simulink model "simulation_model"  (R2024b)
settings: Solver=VariableStepAuto  StartTime=0.0  StopTime=100  MaxStep=1/60  RelTol=1e-3  EnableMultiTasking=on
values from neighbouring files (symbols this model uses):
  c_f = c_f*Cb    [fun00_GFL_pu_2_normial.m]    (also in fun00_GFM_pu_2_normial.m)
  fb = 60    [case_data.m]    (also in sim_m_case1.m; sim_m_case1_bench.m; sim_m_case2.m; sim_m_case2_bench.m)
  ki_i = ki_i_pu*Vb_p_ph/Ib_p_ph    [fun00_GFL_pu_2_normial.m]    (also in fun00_GFM_pu_2_normial.m)
  ki_p = ki_p_pu/Sb*Ib_p_ph    [fun00_GFL_pu_2_normial.m]
  ki_pll = ki_pll/Vb_p_ph    [fun00_GFL_pu_2_normial.m]
  ki_q = ki_q_pu/Sb*Ib_p_ph    [fun00_GFL_pu_2_normial.m]
  kp_i = kp_i_pu*Vb_p_ph/Ib_p_ph    [fun00_GFL_pu_2_normial.m]    (also in fun00_GFM_pu_2_normial.m)
  kp_p = kp_p_pu/Sb*Ib_p_ph    [fun00_GFL_pu_2_normial.m]
  kp_pll = kp_pll/Vb_p_ph    [fun00_GFL_pu_2_normial.m]
  kp_q = kp_q_pu/Sb*Ib_p_ph    [fun00_GFL_pu_2_normial.m]
  l_f = l_f*Lb    [fun00_GFL_pu_2_normial.m]    (also in fun00_GFM_pu_2_normial.m)
  line = mpc.line    [sim_m_case1.m]    (also in sim_m_case1_bench.m; sim_m_case2.m = mpc.line*1.1; sim_m_case2_bench.m = mpc.line*1.1; sim_m_case2_sparse.m = mpc.line*1.1)
  pset = p_set_pu*Sb    [fun00_GFL_pu_2_normial.m]
  qset = q_set_pu*Sb    [fun00_GFL_pu_2_normial.m]
  r_f = r_f*Zb    [fun00_GFL_pu_2_normial.m]    (also in fun00_GFM_pu_2_normial.m)
  Sb = 100*10^6    (= 100000000)    [sim_m_case1.m]    (also in sim_m_case1_bench.m; sim_m_case2.m; sim_m_case2_bench.m; sim_m_case2_sparse.m)
  t_gfl = 35    [sim_m_case1.m]    (also in sim_m_case1_bench.m = 30; sim_m_case2.m; sim_m_case2_bench.m = 30; sim_m_case2_sparse.m)
  t_gfm = 30    [sim_m_case1.m]    (also in sim_m_case1_bench.m; sim_m_case2.m; sim_m_case2_bench.m; sim_m_case2_sparse.m)
  trans_l = mpc.trans_l    [sim_m_case1.m]    (also in sim_m_case1_bench.m; sim_m_case2.m; sim_m_case2_bench.m; sim_m_case2_sparse.m)
  Vb_gfm = 20*10^3    (= 20000)    [sim_m_case1.m]    (also in sim_m_case1_bench.m; sim_m_case2.m; sim_m_case2_bench.m; sim_m_case2_sparse.m)
  Vdc = 3*Vb_p_ph    [fun00_GFL_pu_2_normial.m]    (also in fun00_GFM_pu_2_normial.m)
  wb = 2*pi*fb    (= 376.991118431)    [case_data.m]    (also in sim_m_case1.m; sim_m_case1_bench.m; sim_m_case2.m; sim_m_case2_bench.m)
undefined symbols (not defined in the file or in its folder): c_f_gfm, d_gfl, D_p_gfm, D_p_gfm_s, D_q_gfm, DiscIntNeverNeededParam, Init, Init_GFL, J_gfm, ki_i_gfm, ki_pll_s, ki_vc_gfm, kp_i_gfm, kp_pll_s, kp_vc_gfm, l_f_gfm, P_set_gfm, Q_set_gfm, r_f_gfm, Vb, Vdc_gfm, VSM
libraries: spsThreePhaseVIMeasurementLib x52, spsabctodq0Lib x48, slpidlib x42, spsThreePhaseSeriesRLCBranchLib x27, spsFirstOrderFilterLib x16, spsThreePhaseTransformerTwoWindingsLib x9, spsGroundLib x9, spsPowerPositiveSequenceLib x9, spsdq0toabcLib x9, spsUniversalBridgeLib x9, spsDCVoltageSourceLib x9, spsThreePhaseParallelRLCLoadLib x6
(part 3 of 8)

== system simulation_model/Area 2/INVERTER 6/GFL6 ==
  Cf : spsThreePhaseSeriesRLCBranchLib/Three-Phase Series RLC Branch  Commented=on  LConnTagsString=A|B|C  RConnTagsString=A|B|C  BranchType=C  Resistance=0.1  Inductance=1e-3  Capacitance=RLC_Filter(3)  Measurements=None
  Constant : Constant  Value=Pref
  Constant1 : Constant  Value=Qref
  Display : Display
  Display1 : Display
  Gain : Gain  Gain=1/(Vnom*sqrt(2/3))
  Gain1 : Gain  Gain=1/Sb
  Gain2 : Gain  Gain=1/2/pi/fb
  Gain3 : Gain  Gain=1/Sb
  Ground : spsGroundLib/Ground  Commented=on  LConnTagsString=a
  Measurement : Subsystem
      mask DialogControl ParameterGroupVar Prompt: 参数
  PLL : Subsystem
      mask DialogControl ParameterGroupVar Prompt: 参数
  Subsystem3 : Subsystem
      mask DialogControl ParameterGroupVar Prompt: 参数
  Subsystem4 : Subsystem  mask{Voltage_P=Voltage_P, Voltage_I=Voltage_I, Current_P=Current_P, Current_I=Current_I, Power_P=Power_P, Power_I=Power_I, kf=kf, Dgfl=D_gfl}
      mask prompts: Voltage_P "Voltage Proportional Coefficient"; Voltage_I "Voltage Integral Coefficient"; Current_P "Current Proportional Coefficient"; Current_I "Current Integral Coefficient"; Power_P "Power Proportional Coefficient"; Power_I "Power Integral Coefficient"; kf "Feedforward Coeffcient"; Dgfl "Damping"
      mask DialogControl ParameterGroupVar Prompt: Controller Parameter
  Three-Phase Series RLC Branch : spsThreePhaseSeriesRLCBranchLib/Three-Phase Series RLC Branch  LConnTagsString=A|B|C  RConnTagsString=A|B|C  BranchType=RL  Resistance=RLC_Filter(1)  Inductance=RLC_Filter(2)  Capacitance=1e-6  Measurements=None
  Three-Phase V-I Measurement : spsThreePhaseVIMeasurementLib/Three-Phase V-I Measurement  VoltageMeasurement=phase-to-ground  SetLabelV=off  LabelV=Vabc_s2  Vpu=off  VpuLL=off  CurrentMeasurement=yes  SetLabelI=off  LabelI=Iabc_s2  Ipu=off  Pbase=Pnom  Vbase=Vnom  OutputType=Complex  PhasorSimulation=off  PSBequivalent=0
  Three-Phase V-I Measurement1 : spsThreePhaseVIMeasurementLib/Three-Phase V-I Measurement  VoltageMeasurement=phase-to-ground  SetLabelV=off  LabelV=Vabc_s1  Vpu=off  VpuLL=off  CurrentMeasurement=yes  SetLabelI=off  LabelI=Iabc_s1  Ipu=off  Pbase=Pnom  Vbase=Vnom  OutputType=Complex  PhasorSimulation=off  PSBequivalent=0
  Three-Phase V-I Measurement2 : spsThreePhaseVIMeasurementLib/Three-Phase V-I Measurement  VoltageMeasurement=phase-to-ground  SetLabelV=off  LabelV=Vabc_s0  Vpu=off  VpuLL=off  CurrentMeasurement=yes  SetLabelI=off  LabelI=Iabc_s0  Ipu=off  Pbase=Pnom  Vbase=Vnom  OutputType=Complex  PhasorSimulation=off  PSBequivalent=0
  Three-Phase V-I Measurement3 : spsThreePhaseVIMeasurementLib/Three-Phase V-I Measurement  VoltageMeasurement=phase-to-ground  SetLabelV=off  LabelV=Vabc_s2  Vpu=off  VpuLL=off  CurrentMeasurement=yes  SetLabelI=off  LabelI=Iabc_s2  Ipu=off  Pbase=Pnom  Vbase=Vnom  OutputType=Complex  PhasorSimulation=off  PSBequivalent=0
  Universal Bridge : spsUniversalBridgeLib/Universal Bridge  Arms=3  SnubberResistance=1e5  SnubberCapacitance=inf  Device=Average-model based VSC  Ron=1e-3  Lon=0  ForwardVoltages="[  0  0  ]"  ForwardVoltage=0  GTOparameters=[ 10e-6 , 20e-6 ]  IGBTparameters=[ 1e-6 , 2e-6 ]  Measurements=None  Measurements_2=None  converterType=Rectifier
  Vdc : spsDCVoltageSourceLib/DC Voltage Source  Amplitude=Vdc_nom  Measurements=None
  Vrms : Scope
  a : PMIOPort  Side=Right
  b : PMIOPort  Port=2  Side=Right
  c : PMIOPort  Port=3  Side=Right
  P : Outport
  Omega : Outport  Port=2
  Vabs : Outport  Port=3
  theta_t : Outport  Port=4
  Q : Outport  Port=5
  theta_0 : Outport  Port=6
  wires:
  Measurement/5(Vrms) -> Gain/1, Vrms/1
  Measurement/2(Q) -> Gain1/1, [Q]
  Measurement/3(Vodq) -> [Vodq]
  Measurement/4(Icdq) -> [Icdq]
  [Vabc_s0] -> Measurement/1(Vabc_s0)
  [theta] -> Measurement/4(theta)
  [Iabc_s2] -> Measurement/3(Iabc_s2)
  [Iabc_s0] -> Measurement/2(Iabc_s0)
  [VSG_Uref] -> Universal Bridge/1
  [Vabc_s0] -> PLL/1(Vodq)
  Three-Phase V-I Measurement3/1 -> Subsystem3/1(Vabc)
  Three-Phase V-I Measurement3/2 -> Subsystem3/2(Iabc)
  Subsystem3/1(Vdq0) -> Display/1
  Subsystem3/2(Idq0) -> Display1/1
  PLL/2(theta) -> [theta]
  [Icdq] -> Subsystem4/2(Icdq)
  [Vodq] -> Subsystem4/1(Vodq)
  [theta] -> Subsystem4/3(theta)
  Subsystem4/1(VSG_Uref) -> [VSG_Uref]
  Three-Phase V-I Measurement/1 -> [Vabc_s2]
  Three-Phase V-I Measurement/2 -> [Iabc_s2]
  Three-Phase V-I Measurement2/1 -> [Vabc_s0]
  Three-Phase V-I Measurement2/2 -> [Iabc_s0]
  Three-Phase V-I Measurement1/2 -> [Iabc_s1]
  Three-Phase V-I Measurement1/1 -> [Vabc_s1]
  [P] -> Subsystem4/5(P)
  Constant/1 -> Subsystem4/4(pset)
  Constant1/1 -> Subsystem4/6(qset)
  [theta] -> Subsystem3/3(theta)
  Measurement/1(P) -> Gain3/1, [P]
  PLL/3(Omega) -> [omega], Gain2/1
  Gain/1 -> Vabs/1
  Gain2/1 -> Omega/1
  Gain3/1 -> P/1
  PLL/1(theta_GFL) -> theta_t/1
  Gain1/1 -> Q/1
  PLL/4(theta_0) -> theta_0/1
  [Q] -> Subsystem4/7(Q)
  [omega] -> Subsystem4/8(Omega)
  connections:
  Three-Phase V-I Measurement2/LConn2 -- Cf/LConn2 -- Three-Phase V-I Measurement1/RConn2
  Three-Phase V-I Measurement2/LConn1 -- Cf/LConn1 -- Three-Phase V-I Measurement1/RConn1
  Three-Phase V-I Measurement2/LConn3 -- Cf/LConn3 -- Three-Phase V-I Measurement1/RConn3
  Three-Phase V-I Measurement1/LConn2 -- Three-Phase Series RLC Branch/RConn2
  Three-Phase V-I Measurement1/LConn1 -- Three-Phase Series RLC Branch/RConn1
  Universal Bridge/RConn2 -- Vdc/LConn1
  Vdc/RConn1 -- Universal Bridge/RConn1
  Three-Phase V-I Measurement/LConn3 -- Universal Bridge/LConn3
  Three-Phase V-I Measurement/LConn2 -- Universal Bridge/LConn2
  Three-Phase V-I Measurement/LConn1 -- Universal Bridge/LConn1
  Three-Phase V-I Measurement1/LConn3 -- Three-Phase Series RLC Branch/RConn3
  Three-Phase V-I Measurement2/RConn1 -- a/RConn1
  Three-Phase V-I Measurement2/RConn2 -- b/RConn1
  Three-Phase V-I Measurement2/RConn3 -- c/RConn1
  Three-Phase V-I Measurement3/RConn1 -- Three-Phase Series RLC Branch/LConn1
  Three-Phase Series RLC Branch/LConn2 -- Three-Phase V-I Measurement3/RConn2
  Three-Phase Series RLC Branch/LConn3 -- Three-Phase V-I Measurement3/RConn3
  Three-Phase V-I Measurement3/LConn1 -- Three-Phase V-I Measurement/RConn1
  Three-Phase V-I Measurement3/LConn2 -- Three-Phase V-I Measurement/RConn2
  Three-Phase V-I Measurement3/LConn3 -- Three-Phase V-I Measurement/RConn3
  Ground/LConn1 -- Cf/RConn2 -- Cf/RConn1 -- Cf/RConn3

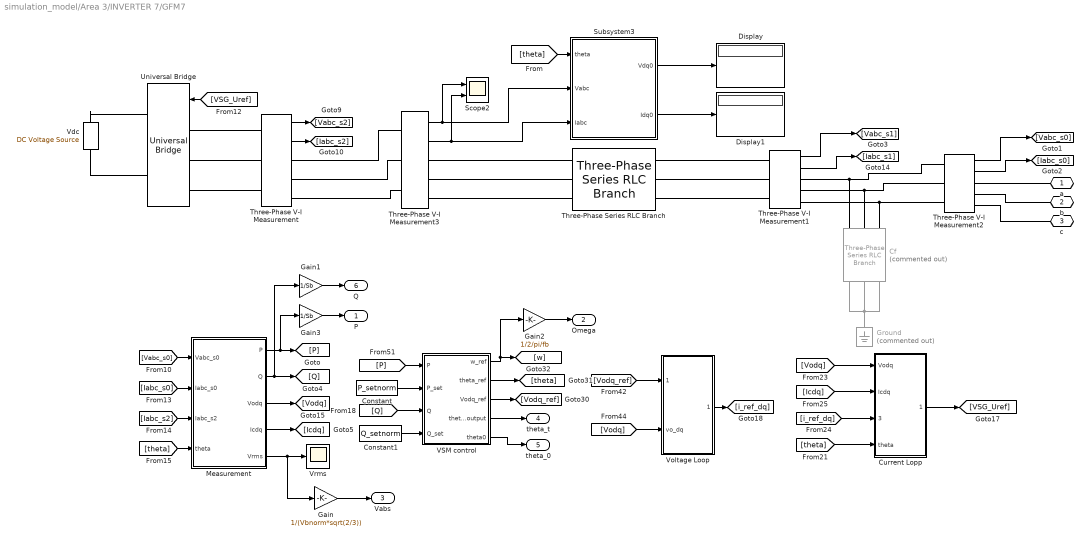
== system simulation_model/Area 3/INVERTER 7/GFM7 ==
  Cf : spsThreePhaseSeriesRLCBranchLib/Three-Phase Series RLC Branch  Commented=on  LConnTagsString=A|B|C  RConnTagsString=A|B|C  BranchType=C  Resistance=0.1  Inductance=1e-3  Capacitance=RLCnorm(3)  Measurements=None
  Constant : Constant  Value=P_setnorm
  Constant1 : Constant  Value=Q_setnorm
  Current Lopp : Subsystem  mask{Current_P=Current_P, Current_I=Current_I}
      mask prompts: Current_P "Current Proportional Coefficient"; Current_I "Current Integral Coefficient"
  Display : Display
  Display1 : Display
  Gain : Gain  Gain=1/(Vbnorm*sqrt(2/3))
  Gain1 : Gain  Gain=1/Sb
  Gain2 : Gain  Gain=1/2/pi/fb
  Gain3 : Gain  Gain=1/Sb
  Ground : spsGroundLib/Ground  Commented=on  LConnTagsString=a
  Measurement : Subsystem
      mask DialogControl ParameterGroupVar Prompt: 参数
  Scope2 : Scope  NumInputPorts=2
  Subsystem3 : Subsystem
      mask DialogControl ParameterGroupVar Prompt: 参数
  Three-Phase Series RLC Branch : spsThreePhaseSeriesRLCBranchLib/Three-Phase Series RLC Branch  LConnTagsString=A|B|C  RConnTagsString=A|B|C  BranchType=RL  Resistance=RLCnorm(1)  Inductance=RLCnorm(2)  Capacitance=1e-6  Measurements=None
  Three-Phase V-I Measurement : spsThreePhaseVIMeasurementLib/Three-Phase V-I Measurement  VoltageMeasurement=phase-to-ground  SetLabelV=off  LabelV=Vabc_s2  Vpu=off  VpuLL=off  CurrentMeasurement=yes  SetLabelI=off  LabelI=Iabc_s2  Ipu=off  Pbase=Pnom  Vbase=Vnom  OutputType=Complex  PhasorSimulation=off  PSBequivalent=0
  Three-Phase V-I Measurement1 : spsThreePhaseVIMeasurementLib/Three-Phase V-I Measurement  VoltageMeasurement=phase-to-ground  SetLabelV=off  LabelV=Vabc_s1  Vpu=off  VpuLL=off  CurrentMeasurement=yes  SetLabelI=off  LabelI=Iabc_s1  Ipu=off  Pbase=Pnom  Vbase=Vnom  OutputType=Complex  PhasorSimulation=off  PSBequivalent=0
  Three-Phase V-I Measurement2 : spsThreePhaseVIMeasurementLib/Three-Phase V-I Measurement  VoltageMeasurement=phase-to-ground  SetLabelV=off  LabelV=Vabc_s0  Vpu=off  VpuLL=off  CurrentMeasurement=yes  SetLabelI=off  LabelI=Iabc_s0  Ipu=off  Pbase=Pnom  Vbase=Vnom  OutputType=Complex  PhasorSimulation=off  PSBequivalent=0
  Three-Phase V-I Measurement3 : spsThreePhaseVIMeasurementLib/Three-Phase V-I Measurement  VoltageMeasurement=phase-to-ground  SetLabelV=off  LabelV=Vabc_s2  Vpu=off  VpuLL=off  CurrentMeasurement=yes  SetLabelI=off  LabelI=Iabc_s2  Ipu=off  Pbase=Pnom  Vbase=Vnom  OutputType=Complex  PhasorSimulation=off  PSBequivalent=0
  Universal Bridge : spsUniversalBridgeLib/Universal Bridge  Arms=3  SnubberResistance=1e5  SnubberCapacitance=inf  Device=Average-model based VSC  Ron=1e-3  Lon=0  ForwardVoltages="[  0  0  ]"  ForwardVoltage=0  GTOparameters=[ 10e-6 , 20e-6 ]  IGBTparameters=[ 1e-6 , 2e-6 ]  Measurements=None  Measurements_2=None  converterType=Rectifier
  VSM control : Subsystem  mask{J=Jnorm, Dp=Dpnorm, Dq=Dqnorm}
      mask prompts: J "Inertia"; Dp "Damping"; Dq "Reactive Droop"
  Vdc : spsDCVoltageSourceLib/DC Voltage Source  Amplitude=Vdcnorm  Measurements=None
  Voltage Loop : Subsystem  mask{Voltage_P=Voltage_P, Voltage_I=Voltage_I}
      mask prompts: Voltage_P "Voltage Proportional Gain"; Voltage_I "Voltage Integral Gain"
  Vrms : Scope
  a : PMIOPort  Side=Right
  b : PMIOPort  Port=2  Side=Right
  c : PMIOPort  Port=3  Side=Right
  P : Outport
  Omega : Outport  Port=2
  Vabs : Outport  Port=3
  theta_t : Outport  Port=4
  theta_0 : Outport  Port=5
  Q : Outport  Port=6
  wires:
  [Vodq_ref] -> Voltage Loop/1(v_ref_dq)
  [Vodq] -> Voltage Loop/2(vo_dq)
  VSM control/2(theta_ref) -> [theta]
  Constant/1 -> VSM control/2(P_set)
  [P] -> VSM control/1(P)
  [Q] -> VSM control/3(Q)
  Three-Phase V-I Measurement1/2 -> [Iabc_s1]
  [VSG_Uref] -> Universal Bridge/1
  Subsystem3/1(Vdq0) -> Display/1
  Three-Phase V-I Measurement2/1 -> [Vabc_s0]
  Three-Phase V-I Measurement/2 -> [Iabc_s2]
  Three-Phase V-I Measurement3/2 -> Scope2/2, Subsystem3/3(Iabc)
  Subsystem3/2(Idq0) -> Display1/1
  Three-Phase V-I Measurement/1 -> [Vabc_s2]
  [theta] -> Subsystem3/1(theta)
  Three-Phase V-I Measurement2/2 -> [Iabc_s0]
  Three-Phase V-I Measurement3/1 -> Scope2/1, Subsystem3/2(Vabc)
  Three-Phase V-I Measurement1/1 -> [Vabc_s1]
  [Vabc_s0] -> Measurement/1(Vabc_s0)
  Measurement/5(Vrms) -> Gain/1, Vrms/1
  Measurement/2(Q) -> Gain1/1, [Q]
  Measurement/4(Icdq) -> [Icdq]
  Measurement/1(P) -> Gain3/1, [P]
  Measurement/3(Vodq) -> [Vodq]
  [theta] -> Measurement/4(theta)
  [Iabc_s2] -> Measurement/3(Iabc_s2)
  [Iabc_s0] -> Measurement/2(Iabc_s0)
  VSM control/3(Vodq_ref) -> [Vodq_ref]
  [Icdq] -> Current Lopp/2(Icdq)
  Current Lopp/1(VSG_Uref) -> [VSG_Uref]
  [Vodq] -> Current Lopp/1(Vodq)
  [theta] -> Current Lopp/4(theta)
  Voltage Loop/1(i_ref_dq) -> [i_ref_dq]
  [i_ref_dq] -> Current Lopp/3(i_ref_dq)
  Constant1/1 -> VSM control/4(Q_set)
  Gain/1 -> Vabs/1
  Gain3/1 -> P/1
  Gain2/1 -> Omega/1
  VSM control/1(w_ref) -> Gain2/1, [w]
  VSM control/4(theta_output) -> theta_t/1
  VSM control/5(theta0) -> theta_0/1
  Gain1/1 -> Q/1
  connections:
  Three-Phase V-I Measurement2/LConn1 -- Cf/LConn1 -- Three-Phase V-I Measurement1/RConn1
  Three-Phase V-I Measurement2/LConn2 -- Cf/LConn2 -- Three-Phase V-I Measurement1/RConn2
  Three-Phase V-I Measurement2/LConn3 -- Cf/LConn3 -- Three-Phase V-I Measurement1/RConn3
  Three-Phase V-I Measurement3/LConn1 -- Three-Phase V-I Measurement/RConn1
  Three-Phase V-I Measurement1/LConn3 -- Three-Phase Series RLC Branch/RConn3
  Three-Phase V-I Measurement2/RConn2 -- b/RConn1
  Three-Phase V-I Measurement/LConn3 -- Universal Bridge/LConn3
  Three-Phase V-I Measurement/LConn1 -- Universal Bridge/LConn1
  Vdc/RConn1 -- Universal Bridge/RConn1
  Three-Phase V-I Measurement2/RConn1 -- a/RConn1
  Three-Phase Series RLC Branch/LConn3 -- Three-Phase V-I Measurement3/RConn3
  Three-Phase V-I Measurement/LConn2 -- Universal Bridge/LConn2
  Three-Phase Series RLC Branch/LConn2 -- Three-Phase V-I Measurement3/RConn2
  Three-Phase V-I Measurement2/RConn3 -- c/RConn1
  Three-Phase V-I Measurement1/LConn1 -- Three-Phase Series RLC Branch/RConn1
  Three-Phase V-I Measurement3/RConn1 -- Three-Phase Series RLC Branch/LConn1
  Universal Bridge/RConn2 -- Vdc/LConn1
  Three-Phase V-I Measurement3/LConn3 -- Three-Phase V-I Measurement/RConn3
  Three-Phase V-I Measurement3/LConn2 -- Three-Phase V-I Measurement/RConn2
  Three-Phase V-I Measurement1/LConn2 -- Three-Phase Series RLC Branch/RConn2
  Cf/RConn3 -- Ground/LConn1 -- Cf/RConn2 -- Cf/RConn1

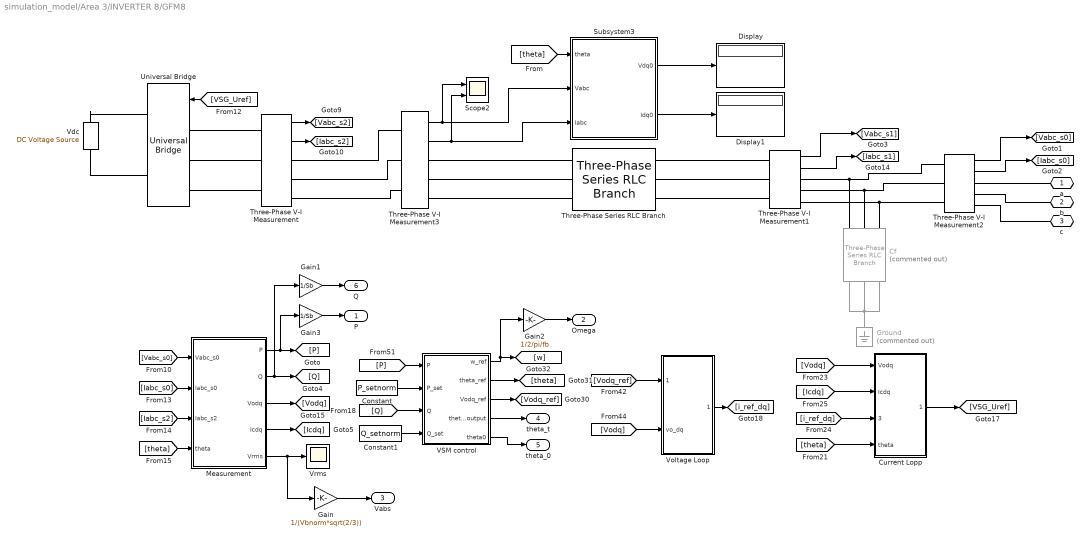
== system simulation_model/Area 3/INVERTER 8/GFM8 ==
  Cf : spsThreePhaseSeriesRLCBranchLib/Three-Phase Series RLC Branch  Commented=on  LConnTagsString=A|B|C  RConnTagsString=A|B|C  BranchType=C  Resistance=0.1  Inductance=1e-3  Capacitance=RLCnorm(3)  Measurements=None
  Constant : Constant  Value=P_setnorm
  Constant1 : Constant  Value=Q_setnorm
  Current Lopp : Subsystem  mask{Current_P=Current_P, Current_I=Current_I}
      mask prompts: Current_P "Current Proportional Coefficient"; Current_I "Current Integral Coefficient"
  Display : Display
  Display1 : Display
  Gain : Gain  Gain=1/(Vbnorm*sqrt(2/3))
  Gain1 : Gain  Gain=1/Sb
  Gain2 : Gain  Gain=1/2/pi/fb
  Gain3 : Gain  Gain=1/Sb
  Ground : spsGroundLib/Ground  Commented=on  LConnTagsString=a
  Measurement : Subsystem
      mask DialogControl ParameterGroupVar Prompt: 参数
  Scope2 : Scope  NumInputPorts=2
  Subsystem3 : Subsystem
      mask DialogControl ParameterGroupVar Prompt: 参数
  Three-Phase Series RLC Branch : spsThreePhaseSeriesRLCBranchLib/Three-Phase Series RLC Branch  LConnTagsString=A|B|C  RConnTagsString=A|B|C  BranchType=RL  Resistance=RLCnorm(1)  Inductance=RLCnorm(2)  Capacitance=1e-6  Measurements=None
  Three-Phase V-I Measurement : spsThreePhaseVIMeasurementLib/Three-Phase V-I Measurement  VoltageMeasurement=phase-to-ground  SetLabelV=off  LabelV=Vabc_s2  Vpu=off  VpuLL=off  CurrentMeasurement=yes  SetLabelI=off  LabelI=Iabc_s2  Ipu=off  Pbase=Pnom  Vbase=Vnom  OutputType=Complex  PhasorSimulation=off  PSBequivalent=0
  Three-Phase V-I Measurement1 : spsThreePhaseVIMeasurementLib/Three-Phase V-I Measurement  VoltageMeasurement=phase-to-ground  SetLabelV=off  LabelV=Vabc_s1  Vpu=off  VpuLL=off  CurrentMeasurement=yes  SetLabelI=off  LabelI=Iabc_s1  Ipu=off  Pbase=Pnom  Vbase=Vnom  OutputType=Complex  PhasorSimulation=off  PSBequivalent=0
  Three-Phase V-I Measurement2 : spsThreePhaseVIMeasurementLib/Three-Phase V-I Measurement  VoltageMeasurement=phase-to-ground  SetLabelV=off  LabelV=Vabc_s0  Vpu=off  VpuLL=off  CurrentMeasurement=yes  SetLabelI=off  LabelI=Iabc_s0  Ipu=off  Pbase=Pnom  Vbase=Vnom  OutputType=Complex  PhasorSimulation=off  PSBequivalent=0
  Three-Phase V-I Measurement3 : spsThreePhaseVIMeasurementLib/Three-Phase V-I Measurement  VoltageMeasurement=phase-to-ground  SetLabelV=off  LabelV=Vabc_s2  Vpu=off  VpuLL=off  CurrentMeasurement=yes  SetLabelI=off  LabelI=Iabc_s2  Ipu=off  Pbase=Pnom  Vbase=Vnom  OutputType=Complex  PhasorSimulation=off  PSBequivalent=0
  Universal Bridge : spsUniversalBridgeLib/Universal Bridge  Arms=3  SnubberResistance=1e5  SnubberCapacitance=inf  Device=Average-model based VSC  Ron=1e-3  Lon=0  ForwardVoltages="[  0  0  ]"  ForwardVoltage=0  GTOparameters=[ 10e-6 , 20e-6 ]  IGBTparameters=[ 1e-6 , 2e-6 ]  Measurements=None  Measurements_2=None  converterType=Rectifier
  VSM control : Subsystem  mask{J=Jnorm, Dp=Dpnorm, Dq=Dqnorm}
      mask prompts: J "Inertia"; Dp "Damping"; Dq "Reactive Droop"
  Vdc : spsDCVoltageSourceLib/DC Voltage Source  Amplitude=Vdcnorm  Measurements=None
  Voltage Loop : Subsystem  mask{Voltage_P=Voltage_P, Voltage_I=Voltage_I}
      mask prompts: Voltage_P "Voltage Proportional Gain"; Voltage_I "Voltage Integral Gain"
  Vrms : Scope
  a : PMIOPort  Side=Right
  b : PMIOPort  Port=2  Side=Right
  c : PMIOPort  Port=3  Side=Right
  P : Outport
  Omega : Outport  Port=2
  Vabs : Outport  Port=3
  theta_t : Outport  Port=4
  theta_0 : Outport  Port=5
  Q : Outport  Port=6
  wires:
  [Vodq_ref] -> Voltage Loop/1(v_ref_dq)
  [Vodq] -> Voltage Loop/2(vo_dq)
  Constant/1 -> VSM control/2(P_set)
  [P] -> VSM control/1(P)
  [Q] -> VSM control/3(Q)
  Three-Phase V-I Measurement1/2 -> [Iabc_s1]
  [VSG_Uref] -> Universal Bridge/1
  Subsystem3/1(Vdq0) -> Display/1
  Three-Phase V-I Measurement2/1 -> [Vabc_s0]
  Three-Phase V-I Measurement/2 -> [Iabc_s2]
  Three-Phase V-I Measurement3/2 -> Scope2/2, Subsystem3/3(Iabc)
  Subsystem3/2(Idq0) -> Display1/1
  Three-Phase V-I Measurement/1 -> [Vabc_s2]
  [theta] -> Subsystem3/1(theta)
  Three-Phase V-I Measurement2/2 -> [Iabc_s0]
  Three-Phase V-I Measurement3/1 -> Scope2/1, Subsystem3/2(Vabc)
  Three-Phase V-I Measurement1/1 -> [Vabc_s1]
  [Vabc_s0] -> Measurement/1(Vabc_s0)
  Measurement/5(Vrms) -> Gain/1, Vrms/1
  Measurement/2(Q) -> Gain1/1, [Q]
  Measurement/4(Icdq) -> [Icdq]
  Measurement/1(P) -> Gain3/1, [P]
  Measurement/3(Vodq) -> [Vodq]
  [theta] -> Measurement/4(theta)
  [Iabc_s2] -> Measurement/3(Iabc_s2)
  [Iabc_s0] -> Measurement/2(Iabc_s0)
  [Icdq] -> Current Lopp/2(Icdq)
  Current Lopp/1(VSG_Uref) -> [VSG_Uref]
  [Vodq] -> Current Lopp/1(Vodq)
  [theta] -> Current Lopp/4(theta)
  Voltage Loop/1(i_ref_dq) -> [i_ref_dq]
  [i_ref_dq] -> Current Lopp/3(i_ref_dq)
  Constant1/1 -> VSM control/4(Q_set)
  Gain/1 -> Vabs/1
  Gain3/1 -> P/1
  Gain2/1 -> Omega/1
  VSM control/1(w_ref) -> Gain2/1, [w]
  VSM control/4(theta_output) -> theta_t/1
  VSM control/5(theta0) -> theta_0/1
  Gain1/1 -> Q/1
  VSM control/3(Vodq_ref) -> [Vodq_ref]
  VSM control/2(theta_ref) -> [theta]
  connections:
  Three-Phase V-I Measurement2/LConn1 -- Cf/LConn1 -- Three-Phase V-I Measurement1/RConn1
  Three-Phase V-I Measurement2/LConn2 -- Cf/LConn2 -- Three-Phase V-I Measurement1/RConn2
  Three-Phase V-I Measurement2/LConn3 -- Cf/LConn3 -- Three-Phase V-I Measurement1/RConn3
  Three-Phase V-I Measurement3/LConn1 -- Three-Phase V-I Measurement/RConn1
  Three-Phase V-I Measurement1/LConn3 -- Three-Phase Series RLC Branch/RConn3
  Three-Phase V-I Measurement2/RConn2 -- b/RConn1
  Three-Phase V-I Measurement/LConn3 -- Universal Bridge/LConn3
  Three-Phase V-I Measurement/LConn1 -- Universal Bridge/LConn1
  Vdc/RConn1 -- Universal Bridge/RConn1
  Three-Phase V-I Measurement2/RConn1 -- a/RConn1
  Three-Phase Series RLC Branch/LConn3 -- Three-Phase V-I Measurement3/RConn3
  Three-Phase V-I Measurement/LConn2 -- Universal Bridge/LConn2
  Three-Phase Series RLC Branch/LConn2 -- Three-Phase V-I Measurement3/RConn2
  Three-Phase V-I Measurement2/RConn3 -- c/RConn1
  Three-Phase V-I Measurement1/LConn1 -- Three-Phase Series RLC Branch/RConn1
  Three-Phase V-I Measurement3/RConn1 -- Three-Phase Series RLC Branch/LConn1
  Universal Bridge/RConn2 -- Vdc/LConn1
  Three-Phase V-I Measurement3/LConn3 -- Three-Phase V-I Measurement/RConn3
  Three-Phase V-I Measurement3/LConn2 -- Three-Phase V-I Measurement/RConn2
  Three-Phase V-I Measurement1/LConn2 -- Three-Phase Series RLC Branch/RConn2
  Cf/RConn3 -- Ground/LConn1 -- Cf/RConn2 -- Cf/RConn1

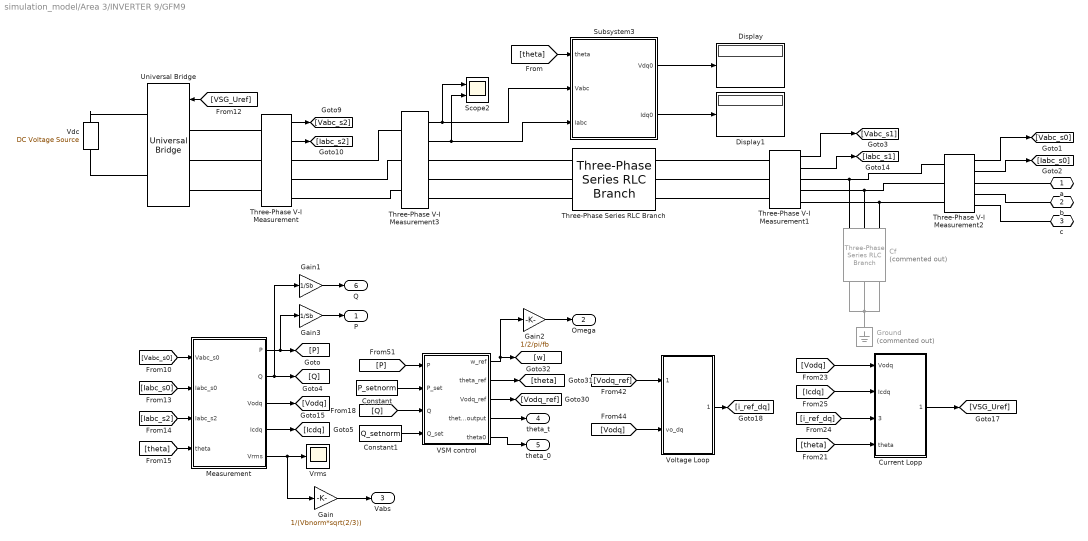
== system simulation_model/Area 3/INVERTER 9/GFM9 ==
  Cf : spsThreePhaseSeriesRLCBranchLib/Three-Phase Series RLC Branch  Commented=on  LConnTagsString=A|B|C  RConnTagsString=A|B|C  BranchType=C  Resistance=0.1  Inductance=1e-3  Capacitance=RLCnorm(3)  Measurements=None
  Constant : Constant  Value=P_setnorm
  Constant1 : Constant  Value=Q_setnorm
  Current Lopp : Subsystem  mask{Current_P=Current_P, Current_I=Current_I}
      mask prompts: Current_P "Current Proportional Coefficient"; Current_I "Current Integral Coefficient"
  Display : Display
  Display1 : Display
  Gain : Gain  Gain=1/(Vbnorm*sqrt(2/3))
  Gain1 : Gain  Gain=1/Sb
  Gain2 : Gain  Gain=1/2/pi/fb
  Gain3 : Gain  Gain=1/Sb
  Ground : spsGroundLib/Ground  Commented=on  LConnTagsString=a
  Measurement : Subsystem
      mask DialogControl ParameterGroupVar Prompt: 参数
  Scope2 : Scope  NumInputPorts=2
  Subsystem3 : Subsystem
      mask DialogControl ParameterGroupVar Prompt: 参数
  Three-Phase Series RLC Branch : spsThreePhaseSeriesRLCBranchLib/Three-Phase Series RLC Branch  LConnTagsString=A|B|C  RConnTagsString=A|B|C  BranchType=RL  Resistance=RLCnorm(1)  Inductance=RLCnorm(2)  Capacitance=1e-6  Measurements=None
  Three-Phase V-I Measurement : spsThreePhaseVIMeasurementLib/Three-Phase V-I Measurement  VoltageMeasurement=phase-to-ground  SetLabelV=off  LabelV=Vabc_s2  Vpu=off  VpuLL=off  CurrentMeasurement=yes  SetLabelI=off  LabelI=Iabc_s2  Ipu=off  Pbase=Pnom  Vbase=Vnom  OutputType=Complex  PhasorSimulation=off  PSBequivalent=0
  Three-Phase V-I Measurement1 : spsThreePhaseVIMeasurementLib/Three-Phase V-I Measurement  VoltageMeasurement=phase-to-ground  SetLabelV=off  LabelV=Vabc_s1  Vpu=off  VpuLL=off  CurrentMeasurement=yes  SetLabelI=off  LabelI=Iabc_s1  Ipu=off  Pbase=Pnom  Vbase=Vnom  OutputType=Complex  PhasorSimulation=off  PSBequivalent=0
  Three-Phase V-I Measurement2 : spsThreePhaseVIMeasurementLib/Three-Phase V-I Measurement  VoltageMeasurement=phase-to-ground  SetLabelV=off  LabelV=Vabc_s0  Vpu=off  VpuLL=off  CurrentMeasurement=yes  SetLabelI=off  LabelI=Iabc_s0  Ipu=off  Pbase=Pnom  Vbase=Vnom  OutputType=Complex  PhasorSimulation=off  PSBequivalent=0
  Three-Phase V-I Measurement3 : spsThreePhaseVIMeasurementLib/Three-Phase V-I Measurement  VoltageMeasurement=phase-to-ground  SetLabelV=off  LabelV=Vabc_s2  Vpu=off  VpuLL=off  CurrentMeasurement=yes  SetLabelI=off  LabelI=Iabc_s2  Ipu=off  Pbase=Pnom  Vbase=Vnom  OutputType=Complex  PhasorSimulation=off  PSBequivalent=0
  Universal Bridge : spsUniversalBridgeLib/Universal Bridge  Arms=3  SnubberResistance=1e5  SnubberCapacitance=inf  Device=Average-model based VSC  Ron=1e-3  Lon=0  ForwardVoltages="[  0  0  ]"  ForwardVoltage=0  GTOparameters=[ 10e-6 , 20e-6 ]  IGBTparameters=[ 1e-6 , 2e-6 ]  Measurements=None  Measurements_2=None  converterType=Rectifier
  VSM control : Subsystem  mask{J=Jnorm, Dp=Dpnorm, Dq=Dqnorm}
      mask prompts: J "Inertia"; Dp "Damping"; Dq "Reactive Droop"
  Vdc : spsDCVoltageSourceLib/DC Voltage Source  Amplitude=Vdcnorm  Measurements=None
  Voltage Loop : Subsystem  mask{Voltage_P=Voltage_P, Voltage_I=Voltage_I}
      mask prompts: Voltage_P "Voltage Proportional Gain"; Voltage_I "Voltage Integral Gain"
  Vrms : Scope
  a : PMIOPort  Side=Right
  b : PMIOPort  Port=2  Side=Right
  c : PMIOPort  Port=3  Side=Right
  P : Outport
  Omega : Outport  Port=2
  Vabs : Outport  Port=3
  theta_t : Outport  Port=4
  theta_0 : Outport  Port=5
  Q : Outport  Port=6
  wires:
  [Vodq_ref] -> Voltage Loop/1(v_ref_dq)
  [Vodq] -> Voltage Loop/2(vo_dq)
  VSM control/2(theta_ref) -> [theta]
  Constant/1 -> VSM control/2(P_set)
  [P] -> VSM control/1(P)
  [Q] -> VSM control/3(Q)
  Three-Phase V-I Measurement1/2 -> [Iabc_s1]
  [VSG_Uref] -> Universal Bridge/1
  Subsystem3/1(Vdq0) -> Display/1
  Three-Phase V-I Measurement2/1 -> [Vabc_s0]
  Three-Phase V-I Measurement/2 -> [Iabc_s2]
  Three-Phase V-I Measurement3/2 -> Scope2/2, Subsystem3/3(Iabc)
  Subsystem3/2(Idq0) -> Display1/1
  Three-Phase V-I Measurement/1 -> [Vabc_s2]
  [theta] -> Subsystem3/1(theta)
  Three-Phase V-I Measurement2/2 -> [Iabc_s0]
  Three-Phase V-I Measurement3/1 -> Scope2/1, Subsystem3/2(Vabc)
  Three-Phase V-I Measurement1/1 -> [Vabc_s1]
  [Vabc_s0] -> Measurement/1(Vabc_s0)
  Measurement/5(Vrms) -> Gain/1, Vrms/1
  Measurement/2(Q) -> Gain1/1, [Q]
  Measurement/4(Icdq) -> [Icdq]
  Measurement/1(P) -> Gain3/1, [P]
  Measurement/3(Vodq) -> [Vodq]
  [theta] -> Measurement/4(theta)
  [Iabc_s2] -> Measurement/3(Iabc_s2)
  [Iabc_s0] -> Measurement/2(Iabc_s0)
  VSM control/3(Vodq_ref) -> [Vodq_ref]
  [Icdq] -> Current Lopp/2(Icdq)
  Current Lopp/1(VSG_Uref) -> [VSG_Uref]
  [Vodq] -> Current Lopp/1(Vodq)
  [theta] -> Current Lopp/4(theta)
  Voltage Loop/1(i_ref_dq) -> [i_ref_dq]
  [i_ref_dq] -> Current Lopp/3(i_ref_dq)
  Constant1/1 -> VSM control/4(Q_set)
  Gain/1 -> Vabs/1
  Gain3/1 -> P/1
  Gain2/1 -> Omega/1
  VSM control/1(w_ref) -> Gain2/1, [w]
  VSM control/5(theta0) -> theta_0/1
  Gain1/1 -> Q/1
  VSM control/4(theta_output) -> theta_t/1
  connections:
  Three-Phase V-I Measurement2/LConn1 -- Cf/LConn1 -- Three-Phase V-I Measurement1/RConn1
  Three-Phase V-I Measurement2/LConn2 -- Cf/LConn2 -- Three-Phase V-I Measurement1/RConn2
  Three-Phase V-I Measurement2/LConn3 -- Cf/LConn3 -- Three-Phase V-I Measurement1/RConn3
  Three-Phase V-I Measurement3/LConn1 -- Three-Phase V-I Measurement/RConn1
  Three-Phase V-I Measurement1/LConn3 -- Three-Phase Series RLC Branch/RConn3
  Three-Phase V-I Measurement2/RConn2 -- b/RConn1
  Three-Phase V-I Measurement/LConn3 -- Universal Bridge/LConn3
  Three-Phase V-I Measurement/LConn1 -- Universal Bridge/LConn1
  Vdc/RConn1 -- Universal Bridge/RConn1
  Three-Phase V-I Measurement2/RConn1 -- a/RConn1
  Three-Phase Series RLC Branch/LConn3 -- Three-Phase V-I Measurement3/RConn3
  Three-Phase V-I Measurement/LConn2 -- Universal Bridge/LConn2
  Three-Phase Series RLC Branch/LConn2 -- Three-Phase V-I Measurement3/RConn2
  Three-Phase V-I Measurement2/RConn3 -- c/RConn1
  Three-Phase V-I Measurement1/LConn1 -- Three-Phase Series RLC Branch/RConn1
  Three-Phase V-I Measurement3/RConn1 -- Three-Phase Series RLC Branch/LConn1
  Universal Bridge/RConn2 -- Vdc/LConn1
  Three-Phase V-I Measurement3/LConn3 -- Three-Phase V-I Measurement/RConn3
  Three-Phase V-I Measurement3/LConn2 -- Three-Phase V-I Measurement/RConn2
  Three-Phase V-I Measurement1/LConn2 -- Three-Phase Series RLC Branch/RConn2
  Cf/RConn3 -- Ground/LConn1 -- Cf/RConn2 -- Cf/RConn1

== system simulation_model/Area 1/INVERTER 1/GFL1/Measurement ==
  Vabc_s0 : Inport
  Iabc_s0 : Inport  Port=2
  Iabc_s2 : Inport  Port=3
  theta : Inport  Port=4
  " " : spsPowerPositiveSequenceLib/Power (Positive-Sequence)  Freq=fb  Vinit=[0, 0]  Iinit=[0, 0]  Ts=0
  Add1 : Sum  Inputs=-+
  Add2 : Sum
  Demux : Demux  Outputs=2
  Demux1 : Demux  Outputs=2
  Fcn : Fcn  Expr=sqrt(u(1)^2 + u(2)^2)
  Gain : Gain
  Gain{1,3..5} (4 alike) : Gain  Gain=3/2
  Gain2 : Gain
  Mux : Mux  Inputs=2
  Mux1 : Mux  Inputs=2
  Mux2 : Mux  Inputs=2
  Product{,1..3} (4 alike) : Product
  Scope{,1..3} (4 alike) : Scope
  Selector : Selector  InputPortWidth=3  IndexOptions=Index vector (dialog)  Indices=[1 2]  OutputSizes=2
  Selector1 : Selector  InputPortWidth=3  IndexOptions=Index vector (dialog)  Indices=[1 2]  OutputSizes=2
  Selector2 : Selector  InputPortWidth=3  IndexOptions=Index vector (dialog)  Indices=[1 2]  OutputSizes=2
  True : Scope
  True P : Scope
  True Q : Scope
  abc to dq0 : spsabctodq0Lib/abc to dq0  Alignment=Aligned with phase A axis
  abc to dq3 : spsabctodq0Lib/abc to dq0  Alignment=Aligned with phase A axis
  abc to dq4 : spsabctodq0Lib/abc to dq0  Alignment=Aligned with phase A axis
  P : Outport
  Q : Outport  Port=2
  Vodq : Outport  Port=3
  Icdq : Outport  Port=4
  Vrms : Outport  Port=5
  wires:
  abc to dq0/1 -> Fcn/1, Selector/1
  theta/1 -> abc to dq4/2, abc to dq3/2, abc to dq0/2
  Add2/1 -> Mux1/2, P/1, Scope2/1
  [Voq] -> Product3/1
  Iabc_s0/1 -> " "/2, abc to dq3/1
  Iabc_s2/1 -> abc to dq4/1
  [Iod] -> Product/2
  [Vod] -> Product1/1
  Selector/1 -> Vodq/1, Demux/1, Scope/1
  [Voq] -> Product2/1
  abc to dq4/1 -> Selector2/1
  [Vod] -> Product/1
  Demux/1 -> [Vod]
  Vabc_s0/1 -> " "/1, abc to dq0/1
  Mux2/1 -> True Q/1
  Fcn/1 -> Vrms/1
  Add1/1 -> Mux2/2, Q/1, Scope3/1
  Mux1/1 -> True P/1
  Selector1/1 -> Demux1/1, Scope1/1
  abc to dq3/1 -> Selector1/1
  Product3/1 -> Gain5/1
  [Ioq] -> Product1/2
  [Iod] -> Product3/2
  Product1/1 -> Gain4/1
  Demux1/2 -> [Ioq]
  Demux1/1 -> [Iod]
  Demux/2 -> [Voq]
  Mux/1 -> True/1
  [Ioq] -> Product2/2
  Selector2/1 -> Icdq/1
  Product2/1 -> Gain3/1
  Product/1 -> Gain1/1
  " "/2 -> Gain2/1
  " "/1 -> Gain/1
  Gain/1 -> Mux1/1, Mux/1
  Gain2/1 -> Mux2/1, Mux/2
  Gain1/1 -> Add2/1
  Gain3/1 -> Add2/2
  Gain4/1 -> Add1/1
  Gain5/1 -> Add1/2

== system simulation_model/Area 1/INVERTER 1/GFL1/PLL ==
  Vodq : Inport
  Clock : Clock
  Constant : Constant  Value=wb
  Constant1 : Constant  Value=2*pi
  Demux : Demux  Outputs=3
  Discrete-Time Integrator : DiscreteIntegrator  SampleTime=-1  ICPrevOutput=DiscIntNeverNeededParam  ICPrevScaledInput=DiscIntNeverNeededParam
  First-Order Filter : spsFirstOrderFilterLib/First-Order Filter  FilterType=Lowpass  Tc=0.08  Ts=0  Initialize=on  Vac_Init=[0, 0, 0]  Vdc_Init=wb  PlotResponse=off  FreqRange="[0,  200,  1]"
  Integrator : Integrator  InitialCondition=InitialV.theta0
  Mod : Math  Operator=mod
  PID Controller1 : slpidlib/PID Controller  Controller=PI  Form=Parallel  TimeDomain=Discrete-time  UseExternalTs=off  SampleTime=-1  IntegratorMethod=Forward Euler  FilterMethod=Forward Euler  ControllerParametersSource=internal  P=PLL_p  I=PLL_i  UseKiTs=off  D=0  UseExternalDerivativeSource=off  N=100  UseFilter=on  TunerSelectOption=Transfer Function Based (PID Tuner App)  InitialConditionSource=internal  InitialConditionForIntegrator=0  InitialConditionForFilter=0  DifferentiatorICPrevScaledInput=0  ExternalReset=none  TrackingMode=off  Kt=1  LimitOutput=off  SatLimitsSource=internal  UpperSaturationLimit=inf  LowerSaturationLimit=-inf  LinearizeAsGain=on  AntiWindupMode=none  Kb=1  LimitIntegrator=off  UpperIntegratorSaturationLimit=inf  LowerIntegratorSaturationLimit=-inf  POutMin=[]  POutMax=[]  IOutMin=[]  IOutMax=[]  DOutMin=[]  DOutMax=[]  NOutMin=[]  NOutMax=[]  SumOutMin=[]  SumOutMax=[]  SaturationOutMin=[]  SaturationOutMax=[]  PParamMin=[]  PParamMax=[]  IParamMin=[]  IParamMax=[]  DParamMin=[]  DParamMax=[]  NParamMin=[]  NParamMax=[]  KbParamMin=[]  KbParamMax=[]  KtParamMin=[]  KtParamMax=[]  KbOutMin=[]  KbOutMax=[]  KtOutMin=[]  KtOutMax=[]  IntegratorOutMin=[]  IntegratorOutMax=[]  FilterOutMin=[]  FilterOutMax=[]  SumI1OutMin=[]  SumI1OutMax=[]  SumI2OutMin=[]  SumI2OutMax=[]  SumI3OutMin=[]  SumI3OutMax=[]  SumI4OutMin=[]  SumI4OutMax=[]  SumDOutMin=[]  SumDOutMax=[]  DifferentiatorOutMin=[]  DifferentiatorOutMax=[]  FilterDiffOutCoefMin=[]  FilterDiffOutCoefMax=[]  ReciprocalOutMin=[]  ReciprocalOutMax=[]  SumDenOutMin=[]  SumDenOutMax=[]  SumNumOutMin=[]  SumNumOutMax=[]  DivideOutMin=[]  DivideOutMax=[]  UdiffTsProdOutMin=[]  UdiffTsProdOutMax=[]  NTsProdOutMin=[]  NTsProdOutMax=[]  UintegralTsProdOutMin=[]  UintegralTsProdOutMax=[]  UngainTsProdOutMin=[]  UngainTsProdOutMax=[]  ClampingZeroOutDataTypeStr=Inherit: Inherit via back propagation  ClampingZeroOutMin=[]  ClampingZeroOutMax=[]  FilterDenConstantOutDataTypeStr=Inherit: Inherit via back propagation  FilterDenConstantOutMin=[]  FilterDenConstantOutMax=[]  PCopyOutDataTypeStr=Inherit: Inherit via back propagation  PCopyOutMin=[]  PCopyOutMax=[]  NCopyOutDataTypeStr=Inherit: Inherit via back propagation  NCopyOutMin=[]  NCopyOutMax=[]  IntegratorContinuousStateAttributes=''  IntegratorStateMustResolveToSignalObject=off  IntegratorRTWStateStorageClass=Auto  FilterContinuousStateAttributes=''  FilterStateMustResolveToSignalObject=off  FilterRTWStateStorageClass=Auto  ParallelPVariant=InternalParameters  IdealPVariant=Disabled  IVariant=InternalParameters  DVariant=Disabled  IntegratorVariant=Discrete  SatVariant=Disabled  AWVariant=Passthrough  PCopyVariant=Disabled  TRVariant=Disabled  FdbkBlocksVariant=Forward  IdealPFdbkVariant=Disabled  SatFdbkVariant=Disabled  DerivativeFilterVariant=Disabled  NVariant=Disabled  NCopyVariant=Disabled_SignalSpec  FilterICVariant=Disabled  IntegratorICVariant=InternalICs  ExternalResetVariant=Disabled  TRSumVariant=Passthrough  SumFdbkVariant=Disabled  SumVariant=Sum_PI  TsampFilterVariant=InternalTs  TsampNgainVariant=Passthrough  TsampIntegralVariant=Disabled_SignalSpec  ExternalSaturationOutDataTypeStr=Inherit: Same as second input  DerivativeSourceVariant=Disabled  PreIntVariant=InternalPreInt
  PID Controller2 : slpidlib/PID Controller  Controller=PI  Form=Parallel  TimeDomain=Discrete-time  UseExternalTs=off  SampleTime=-1  IntegratorMethod=Forward Euler  FilterMethod=Forward Euler  ControllerParametersSource=internal  P=kp_pll_s(1)  I=ki_pll_s(1)  UseKiTs=off  D=0  UseExternalDerivativeSource=off  N=100  UseFilter=on  TunerSelectOption=Transfer Function Based (PID Tuner App)  InitialConditionSource=internal  InitialConditionForIntegrator=0  InitialConditionForFilter=0  DifferentiatorICPrevScaledInput=0  ExternalReset=none  TrackingMode=off  Kt=1  LimitOutput=off  SatLimitsSource=internal  UpperSaturationLimit=inf  LowerSaturationLimit=-inf  LinearizeAsGain=on  AntiWindupMode=none  Kb=1  LimitIntegrator=off  UpperIntegratorSaturationLimit=inf  LowerIntegratorSaturationLimit=-inf  POutMin=[]  POutMax=[]  IOutMin=[]  IOutMax=[]  DOutMin=[]  DOutMax=[]  NOutMin=[]  NOutMax=[]  SumOutMin=[]  SumOutMax=[]  SaturationOutMin=[]  SaturationOutMax=[]  PParamMin=[]  PParamMax=[]  IParamMin=[]  IParamMax=[]  DParamMin=[]  DParamMax=[]  NParamMin=[]  NParamMax=[]  KbParamMin=[]  KbParamMax=[]  KtParamMin=[]  KtParamMax=[]  KbOutMin=[]  KbOutMax=[]  KtOutMin=[]  KtOutMax=[]  IntegratorOutMin=[]  IntegratorOutMax=[]  FilterOutMin=[]  FilterOutMax=[]  SumI1OutMin=[]  SumI1OutMax=[]  SumI2OutMin=[]  SumI2OutMax=[]  SumI3OutMin=[]  SumI3OutMax=[]  SumI4OutMin=[]  SumI4OutMax=[]  SumDOutMin=[]  SumDOutMax=[]  DifferentiatorOutMin=[]  DifferentiatorOutMax=[]  FilterDiffOutCoefMin=[]  FilterDiffOutCoefMax=[]  ReciprocalOutMin=[]  ReciprocalOutMax=[]  SumDenOutMin=[]  SumDenOutMax=[]  SumNumOutMin=[]  SumNumOutMax=[]  DivideOutMin=[]  DivideOutMax=[]  UdiffTsProdOutMin=[]  UdiffTsProdOutMax=[]  NTsProdOutMin=[]  NTsProdOutMax=[]  UintegralTsProdOutMin=[]  UintegralTsProdOutMax=[]  UngainTsProdOutMin=[]  UngainTsProdOutMax=[]  ClampingZeroOutDataTypeStr=Inherit: Inherit via back propagation  ClampingZeroOutMin=[]  ClampingZeroOutMax=[]  FilterDenConstantOutDataTypeStr=Inherit: Inherit via back propagation  FilterDenConstantOutMin=[]  FilterDenConstantOutMax=[]  PCopyOutDataTypeStr=Inherit: Inherit via back propagation  PCopyOutMin=[]  PCopyOutMax=[]  NCopyOutDataTypeStr=Inherit: Inherit via back propagation  NCopyOutMin=[]  NCopyOutMax=[]  IntegratorContinuousStateAttributes=''  IntegratorStateMustResolveToSignalObject=off  IntegratorRTWStateStorageClass=Auto  FilterContinuousStateAttributes=''  FilterStateMustResolveToSignalObject=off  FilterRTWStateStorageClass=Auto  ParallelPVariant=InternalParameters  IdealPVariant=Disabled  IVariant=InternalParameters  DVariant=Disabled  IntegratorVariant=Discrete  SatVariant=Disabled  AWVariant=Passthrough  PCopyVariant=Disabled  TRVariant=Disabled  FdbkBlocksVariant=Forward  IdealPFdbkVariant=Disabled  SatFdbkVariant=Disabled  DerivativeFilterVariant=Disabled  NVariant=Disabled  NCopyVariant=Disabled_SignalSpec  FilterICVariant=Disabled  IntegratorICVariant=InternalICs  ExternalResetVariant=Disabled  TRSumVariant=Passthrough  SumFdbkVariant=Disabled  SumVariant=Sum_PI  TsampFilterVariant=InternalTs  TsampNgainVariant=Passthrough  TsampIntegralVariant=Disabled_SignalSpec  ExternalSaturationOutDataTypeStr=Inherit: Same as second input  DerivativeSourceVariant=Disabled  PreIntVariant=InternalPreInt
  Scope : Scope
  Sum : Sum  Inputs=|++
  Switch : Switch  Threshold=t_gfl  SaturateOnIntegerOverflow=off  InputSameDT=off
  Terminator : Terminator
  Terminator1 : Terminator
  abc to dq3 : spsabctodq0Lib/abc to dq0  Alignment=Aligned with phase A axis
  theta_GFL : Outport
  theta : Outport  Port=2
  Omega : Outport  Port=3
  theta_0 : Outport  Port=4
  wires:
  abc to dq3/1 -> Demux/1
  Constant/1 -> Sum/2
  Integrator/1 -> theta_GFL/1, Mod/1, abc to dq3/2
  [pll_output] -> Discrete-Time Integrator/1, Sum/1
  Vodq/1 -> abc to dq3/1
  Demux/2 -> [pll_input]
  Demux/3 -> Terminator/1
  Demux/1 -> Terminator1/1
  Constant1/1 -> Mod/2
  Mod/1 -> Scope/1, theta/1
  First-Order Filter/1 -> Omega/1, Integrator/1
  Discrete-Time Integrator/1 -> theta_0/1
  [pll_input] -> PID Controller2/1
  Clock/1 -> Switch/2
  [pll_input] -> PID Controller1/1
  PID Controller1/1 -> Switch/3
  PID Controller2/1 -> Switch/1
  Switch/1 -> [pll_output]
  Sum/1 -> First-Order Filter/1

== system simulation_model/Area 1/INVERTER 1/GFL1/Subsystem3 ==
  Vabc : Inport
  Iabc : Inport  Port=2
  theta : Inport  Port=3
  Scope : Scope
  abc to dq1 : spsabctodq0Lib/abc to dq0  Alignment=Aligned with phase A axis
  abc to dq2 : spsabctodq0Lib/abc to dq0  Alignment=Aligned with phase A axis
  Vdq0 : Outport
  Idq0 : Outport  Port=2
  wires:
  Iabc/1 -> abc to dq2/1
  abc to dq1/1 -> Vdq0/1
  Vabc/1 -> abc to dq1/1
  abc to dq2/1 -> Scope/1, Idq0/1
  theta/1 -> abc to dq2/2, abc to dq1/2
